simulink model "Capacitor"  (R2021a)
settings: Solver=VariableStepAuto  StartTime=0.0  StopTime=10.0  RelTol=1e-3
settings Model: Creator=Admin  LastModifiedBy=Admin

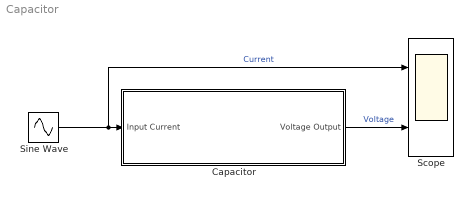
== system Capacitor ==
  Capacitor : Subsystem
  Scope : Scope  NumInputPorts=2
  Sine Wave : Sin  SampleTime=0
  wires:
  Sine Wave/1 -> Scope/1, Capacitor/1(Input Current)  "Current"
  Capacitor/1(Voltage Output) -> Scope/2  "Voltage"

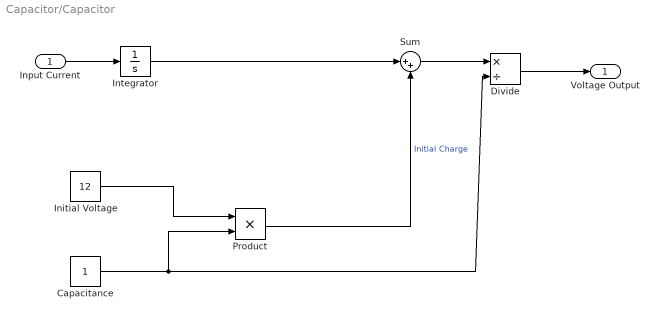
== system Capacitor/Capacitor ==
  Input Current : Inport
  Capacitance : Constant
  Divide : Product  Inputs=*/
  Initial Voltage : Constant  Value=12
  Integrator : Integrator
  Product : Product
  Sum : Sum  Inputs=|++
  Voltage Output : Outport
  wires:
  Input Current/1 -> Integrator/1
  Integrator/1 -> Sum/1
  Sum/1 -> Divide/1
  Divide/1 -> Voltage Output/1
  Initial Voltage/1 -> Product/1
  Capacitance/1 -> Product/2, Divide/2
  Product/1 -> Sum/2  "Initial Charge"
